simulink model "Malha_de_Controle_Drone"  (R2016a)
settings: Solver=VariableStepAuto  SolverMode=SingleTasking  StartTime=0.0  StopTime=60  RelTol=1e-3
values from neighbouring files (symbols this model uses):
  chave_circular = 0    [Controle_LQR_ARDrone.m]    (also in Controle_LQR_Robusto_Drone.m)
  chave_oito = 1    [Controle_LQR_ARDrone.m]    (also in Controle_LQR_Robusto_Drone.m)
  Cx = 0.3    [Controle_LQR_ARDrone.m]    (also in Controle_LQR_Robusto_Drone.m; TesteDeRobustez.m = 1)
  Cy = 0.1    [Controle_LQR_ARDrone.m]    (also in Controle_LQR_Robusto_Drone.m; TesteDeRobustez.m = 3)
  fimax = 0.26    [Controle_LQR_ARDrone.m]    (also in Controle_LQR_Robusto_Drone.m = 0.45)
  g = 9.8    [Controle_LQR_ARDrone.m]    (also in Controle_LQR_Robusto_Drone.m)
  K_psi = K_psi2(:,1:2)    [Controle_LQR_ARDrone.m]    (also in Controle_LQR_Robusto_Drone.m)
  K_z = K_z2(:,1:2)    [Controle_LQR_ARDrone.m]    (also in Controle_LQR_Robusto_Drone.m)
  Kfi_y = Kfi_y2(:,1:4)    [Controle_LQR_ARDrone.m]    (also in Controle_LQR_Robusto_Drone.m)
  Ki_fi_y = Kfi_y2(:,5)    [Controle_LQR_ARDrone.m]    (also in Controle_LQR_Robusto_Drone.m)
  Ki_psi = K_psi2(:,3)    [Controle_LQR_ARDrone.m]    (also in Controle_LQR_Robusto_Drone.m)
  Ki_theta_x = Ktheta_x2(:,5)    [Controle_LQR_ARDrone.m]    (also in Controle_LQR_Robusto_Drone.m)
  Ki_z = K_z2(:,3)    [Controle_LQR_ARDrone.m]    (also in Controle_LQR_Robusto_Drone.m)
  Kpsi = 1    [Controle_LQR_ARDrone.m]    (also in Controle_LQR_Robusto_Drone.m)
  Ktheta_x = Ktheta_x2(:,1:4)    [Controle_LQR_ARDrone.m]    (also in Controle_LQR_Robusto_Drone.m)
  Kz = 1.3    [Controle_LQR_ARDrone.m]    (also in Controle_LQR_Robusto_Drone.m)
  psimax = 1.74    [Controle_LQR_ARDrone.m]    (also in Controle_LQR_Robusto_Drone.m = 5.15)
  thetamax = 0.26    [Controle_LQR_ARDrone.m]    (also in Controle_LQR_Robusto_Drone.m = 0.52)
  tpsi = 0.3    [Controle_LQR_ARDrone.m]    (also in Controle_LQR_Robusto_Drone.m; TesteDeRobustez.m = 0.4)
  tz = 0.4    [Controle_LQR_ARDrone.m]    (also in Controle_LQR_Robusto_Drone.m; TesteDeRobustez.m = 0.8)
  wfi = 4.47    [Controle_LQR_ARDrone.m]    (also in Controle_LQR_Robusto_Drone.m)
  wtheta = 4.47    [Controle_LQR_ARDrone.m]    (also in Controle_LQR_Robusto_Drone.m)
  zetafi = 0.5    [Controle_LQR_ARDrone.m]    (also in Controle_LQR_Robusto_Drone.m)
  zetatheta = 0.5    [Controle_LQR_ARDrone.m]    (also in Controle_LQR_Robusto_Drone.m)
  zmax = 1.0    (= 1)    [Controle_LQR_ARDrone.m]    (also in Controle_LQR_Robusto_Drone.m = 2)
settings Model: Creator=root  LastModifiedBy=JesseAlves
settings DebuggingCC: SFUnexpectedBacktrackingDiag=error  SFNoUnconditionalDefaultTransitionDiag=error
settings SFSimCC: SimUseLocalCustomCode=on
settings RTWCC: RTWUseLocalCustomCode=on
settings GRTTargetCC: TargetLangStandard=C99 (ISO)  GeneratePreprocessorConditionals=Use local settings
settings ConfigComp: CovMetricSettings=dwe  CovHtmlReporting=off  CovSaveCumulativeToWorkspaceVar=off  CovSaveSingleToWorkspaceVar=off  CovModelRefEnable=Off  CovExternalEMLEnable=on

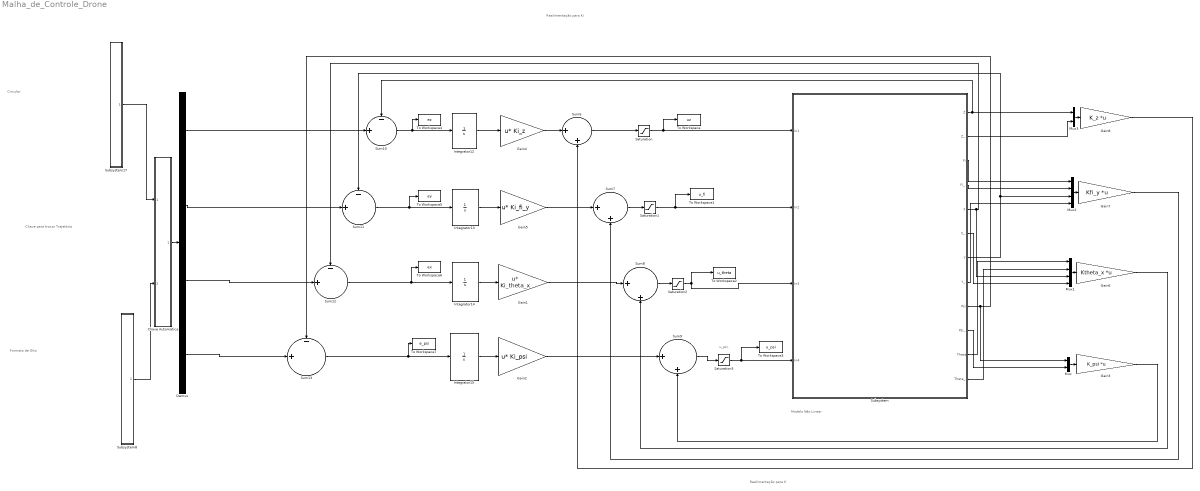
== system Malha_de_Controle_Drone ==
  note: Chave para
      | trocar Trajetória
  note: u_psi.
  note: Realimentação para Ki
  note: Modelo Não Linear
  note: Circular
  note: Formato
      | de Oito
  note: Realimentação para K
  Chave Automática : Subsystem
  Demux : Demux
  Gain1 : Gain  Gain=Ki_theta_x  Multiplication=Matrix(u*K)
  Gain2 : Gain  Gain=Ki_psi  Multiplication=Matrix(u*K)
  Gain3 : Gain  Gain=K_psi  Multiplication=Matrix(K*u)
  Gain4 : Gain  Gain=Ki_z  Multiplication=Matrix(u*K)
  Gain5 : Gain  Gain=Ki_fi_y  Multiplication=Matrix(u*K)
  Gain6 : Gain  Gain=Ktheta_x  Multiplication=Matrix(K*u)
  Gain7 : Gain  Gain=Kfi_y  Multiplication=Matrix(K*u)
  Gain8 : Gain  Gain=K_z  Multiplication=Matrix(K*u)
  Integrator{12..15} (4 alike) : Integrator
  Mux : Mux  Inputs=2
  Mux1 : Mux
  Mux2 : Mux
  Mux3 : Mux  Inputs=2
  Saturation{,1..3} (4 alike) : Saturate  UpperLimit=1  LowerLimit=-1
  Subsystem : Subsystem
  Subsystem17 : Subsystem
  Subsystem8 : Subsystem
  Sum{10..13} (4 alike) : Sum  Inputs=-+|
  Sum{6..9} (4 alike) : Sum  Inputs=|++
  To Workspace : ToWorkspace  VariableName=uz  SampleTime=-1
  To Workspace1 : ToWorkspace  VariableName=u_fi  SampleTime=-1
  To Workspace2 : ToWorkspace  VariableName=u_theta  SampleTime=-1
  To Workspace3 : ToWorkspace  VariableName=u_psi  SampleTime=-1
  To Workspace4 : ToWorkspace  VariableName=ez  SampleTime=-1
  To Workspace5 : ToWorkspace  VariableName=ey  SampleTime=-1
  To Workspace6 : ToWorkspace  VariableName=ex  SampleTime=-1
  To Workspace7 : ToWorkspace  VariableName=e_psi  SampleTime=-1
  wires:
  Sum6/1 -> Saturation/1
  Sum7/1 -> Saturation1/1
  Sum8/1 -> Saturation2/1
  Sum9/1 -> Saturation3/1
  Saturation/1 -> To Workspace/1, Subsystem/1(In1)
  Saturation1/1 -> To Workspace1/1, Subsystem/2(In2)
  Saturation2/1 -> To Workspace2/1, Subsystem/3(In3)
  Saturation3/1 -> To Workspace3/1, Subsystem/4(In4)
  Demux/1 -> Sum10/2
  Demux/2 -> Sum11/2
  Demux/3 -> Sum12/2
  Demux/4 -> Sum13/2
  Sum10/1 -> To Workspace4/1, Integrator12/1
  Integrator12/1 -> Gain4/1
  Sum11/1 -> To Workspace5/1, Integrator13/1
  Integrator13/1 -> Gain5/1
  Sum12/1 -> To Workspace6/1, Integrator14/1
  Integrator14/1 -> Gain1/1
  Integrator15/1 -> Gain2/1
  Sum13/1 -> To Workspace7/1, Integrator15/1
  Gain4/1 -> Sum6/1
  Gain5/1 -> Sum7/1
  Gain1/1 -> Sum8/1
  Gain2/1 -> Sum9/1
  Subsystem17/1(Out1) -> Chave Automática/1(In1)
  Subsystem8/1(Out1) -> Chave Automática/2(In2)
  Chave Automática/1(Out1) -> Demux/1
  Subsystem/9(Psi) -> Mux/1, Sum13/1
  Mux/1 -> Gain3/1
  Subsystem/10(Psi_.) -> Mux/2
  Gain3/1 -> Sum9/2
  Mux1/1 -> Gain6/1
  Subsystem/11(Theta) -> Mux1/1
  Subsystem/12(Theta_.) -> Mux1/2
  Subsystem/5(X) -> Sum12/1, Mux1/3
  Subsystem/6(X_.) -> Mux1/4
  Gain6/1 -> Sum8/2
  Subsystem/3(Fi) -> Mux2/1
  Subsystem/4(Fi_.) -> Mux2/2
  Subsystem/7("Y ") -> Mux2/3, Sum11/1
  Subsystem/8(Y_.) -> Mux2/4
  Mux2/1 -> Gain7/1
  Gain7/1 -> Sum7/2
  Subsystem/1(Z) -> Sum10/1, Mux3/1
  Subsystem/2("Z_. ") -> Mux3/2
  Mux3/1 -> Gain8/1
  Gain8/1 -> Sum6/2

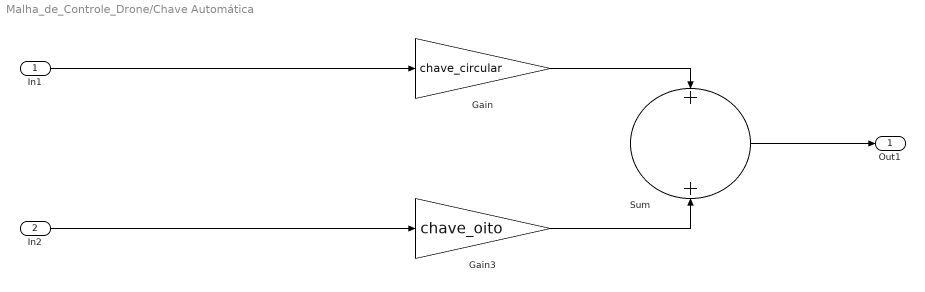
== system Malha_de_Controle_Drone/Chave Automática ==
  In1 : Inport
  In2 : Inport  Port=2
  Gain : Gain  Gain=chave_circular
  Gain3 : Gain  Gain=chave_oito
  Sum : Sum  Inputs=+|+
  Out1 : Outport
  wires:
  Sum/1 -> Out1/1
  In1/1 -> Gain/1
  In2/1 -> Gain3/1
  Gain3/1 -> Sum/2
  Gain/1 -> Sum/1

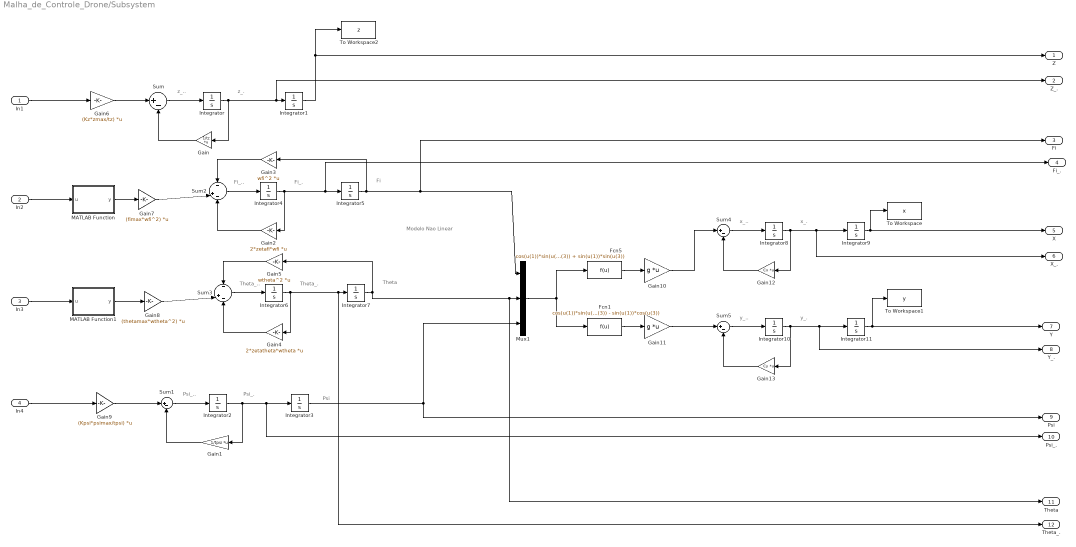
== system Malha_de_Controle_Drone/Subsystem ==
  note: Modelo Nao Linear
  note: z_..
  note: z_.
  note: Psi
  note: Psi_.
  note: Psi_..
  note: Fi
  note: Fi_.
  note: Fi_..
  note: Theta_..
  note: Theta_.
  note: Theta
  note: x_.
  note: x_..
  note: y_.
  note: y_..
  In1 : Inport
  In2 : Inport  Port=2
  In3 : Inport  Port=3
  In4 : Inport  Port=4
  Fcn1 : Fcn  Expr=cos(u(1))*sin(u(2))*sin(u(3)) - sin(u(1))*cos(u(3))
  Fcn5 : Fcn  Expr=cos(u(1))*sin(u(2))*cos(u(3)) + sin(u(1))*sin(u(3))
  Gain : Gain  Gain=1/tz  Multiplication=Matrix(K*u)
  Gain1 : Gain  Gain=1/tpsi  Multiplication=Matrix(K*u)
  Gain10 : Gain  Gain=g  Multiplication=Matrix(K*u)
  Gain11 : Gain  Gain=g  Multiplication=Matrix(K*u)
  Gain12 : Gain  Gain=Cx  Multiplication=Matrix(K*u)
  Gain13 : Gain  Gain=Cy  Multiplication=Matrix(K*u)
  Gain2 : Gain  Gain=2*zetafi*wfi  Multiplication=Matrix(K*u)
  Gain3 : Gain  Gain=wfi^2  Multiplication=Matrix(K*u)
  Gain4 : Gain  Gain=2*zetatheta*wtheta  Multiplication=Matrix(K*u)
  Gain5 : Gain  Gain=wtheta^2  Multiplication=Matrix(K*u)
  Gain6 : Gain  Gain=(Kz*zmax/tz)  Multiplication=Matrix(K*u)
  Gain7 : Gain  Gain=(fimax*wfi^2)  Multiplication=Matrix(K*u)
  Gain8 : Gain  Gain=(thetamax*wtheta^2)  Multiplication=Matrix(K*u)
  Gain9 : Gain  Gain=(Kpsi*psimax/tpsi)  Multiplication=Matrix(K*u)
  Integrator{,1..11} (12 alike) : Integrator
  MATLAB Function : MATLAB Function  TreatAsAtomicUnit=on
  MATLAB Function1 : MATLAB Function  TreatAsAtomicUnit=on
  Mux1 : Mux  Inputs=3
  Sum{,1,4..5} (4 alike) : Sum  Inputs=|+-
  Sum2 : Sum  Inputs=-|+-
  Sum3 : Sum  Inputs=-|+-
  To Workspace : ToWorkspace  VariableName=x  SampleTime=-1
  To Workspace1 : ToWorkspace  VariableName=y  SampleTime=-1
  To Workspace2 : ToWorkspace  VariableName=z  SampleTime=-1
  Z : Outport
  "Z_. " : Outport  Port=2
  Fi : Outport  Port=3
  Fi_. : Outport  Port=4
  X : Outport  Port=5
  X_. : Outport  Port=6
  "Y " : Outport  Port=7
  Y_. : Outport  Port=8
  Psi : Outport  Port=9
  Psi_. : Outport  Port=10
  Theta : Outport  Port=11
  Theta_. : Outport  Port=12
  wires:
  Integrator11/1 -> To Workspace1/1, "Y "/1
  Gain11/1 -> Sum5/1
  Gain8/1 -> Sum3/2
  Gain4/1 -> Sum3/3
  Sum5/1 -> Integrator10/1
  Sum2/1 -> Integrator4/1
  MATLAB Function1/1(y) -> Gain8/1
  Sum3/1 -> Integrator6/1
  Gain/1 -> Sum/2
  Gain7/1 -> Sum2/2
  Gain6/1 -> Sum/1
  Sum4/1 -> Integrator8/1
  Integrator1/1 -> To Workspace2/1, Z/1
  Fcn5/1 -> Gain10/1
  Integrator3/1 -> Psi/1, Mux1/3
  Integrator5/1 -> Fi/1, Mux1/1, Gain3/1
  Fcn1/1 -> Gain11/1
  Integrator4/1 -> Fi_./1, Integrator5/1, Gain2/1
  Gain5/1 -> Sum3/1
  Integrator2/1 -> Psi_./1, Integrator3/1, Gain1/1
  Integrator/1 -> "Z_. "/1, Integrator1/1, Gain/1
  Gain1/1 -> Sum1/2
  Integrator6/1 -> Theta_./1, Integrator7/1, Gain4/1
  Gain2/1 -> Sum2/3
  Gain3/1 -> Sum2/1
  Integrator9/1 -> To Workspace/1, X/1
  Gain10/1 -> Sum4/1
  Integrator10/1 -> Y_./1, Integrator11/1, Gain13/1
  Integrator7/1 -> Theta/1, Mux1/2, Gain5/1
  Gain13/1 -> Sum5/2
  Mux1/1 -> Fcn1/1, Fcn5/1
  Gain12/1 -> Sum4/2
  Sum1/1 -> Integrator2/1
  Gain9/1 -> Sum1/1
  Sum/1 -> Integrator/1
  MATLAB Function/1(y) -> Gain7/1
  Integrator8/1 -> X_./1, Integrator9/1, Gain12/1
  In1/1 -> Gain6/1
  In2/1 -> MATLAB Function/1(u)
  In3/1 -> MATLAB Function1/1(u)
  In4/1 -> Gain9/1

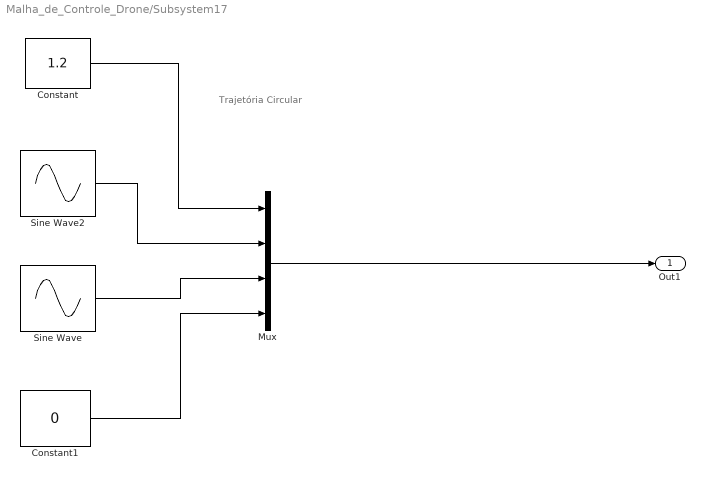
== system Malha_de_Controle_Drone/Subsystem17 ==
  note: Trajetória Circular
  Constant : Constant  Value=1.2
  Constant1 : Constant  Value=0
  Mux : Mux
  Sine Wave : Sin  Frequency=0.8  SampleTime=0
  Sine Wave2 : Sin  Frequency=0.8  Phase=pi/2  SampleTime=0
  Out1 : Outport
  wires:
  Mux/1 -> Out1/1
  Constant/1 -> Mux/1
  Sine Wave2/1 -> Mux/2
  Sine Wave/1 -> Mux/3
  Constant1/1 -> Mux/4

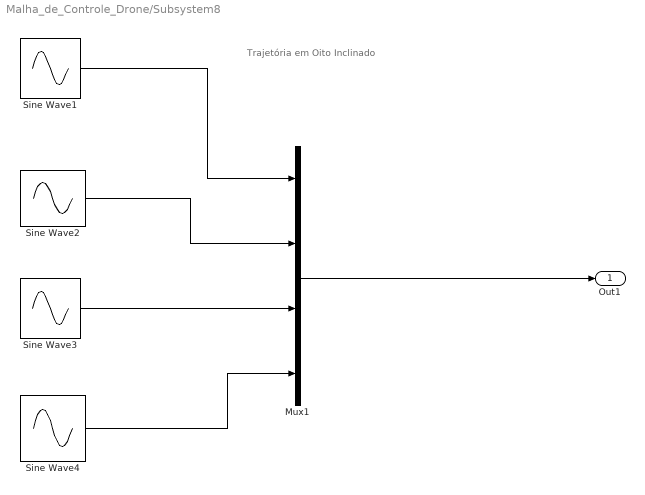
== system Malha_de_Controle_Drone/Subsystem8 ==
  note: Trajetória em Oito Inclinado
  Mux1 : Mux
  Sine Wave1 : Sin  Amplitude=0.5  Bias=1.2  Frequency=0.4  SampleTime=0
  Sine Wave2 : Sin  Frequency=0.4  SampleTime=0
  Sine Wave3 : Sin  Amplitude=0.5  Frequency=0.8  SampleTime=0
  Sine Wave4 : Sin  Amplitude=-pi/6  Frequency=0.4  SampleTime=0
  Out1 : Outport
  wires:
  Mux1/1 -> Out1/1
  Sine Wave1/1 -> Mux1/1
  Sine Wave2/1 -> Mux1/2
  Sine Wave3/1 -> Mux1/3
  Sine Wave4/1 -> Mux1/4

== matlab function Malha_de_Controle_Drone/Subsystem/MATLAB Function1 ==
  data: u input; y output
% ==> Funcao para calcular valor de K_fi
function y = k_theta(u)
    k_theta_min = 1;
    k_theta_max = 2;
    
    if abs(u) > 0.5
        u = k_theta_min*u;
    else       
        u = k_theta_max*u;
    end
y = u;

== matlab function Malha_de_Controle_Drone/Subsystem/MATLAB Function ==
  data: u input; y output
% ==> Funcao para calcular valor de K_fi
function y = k_fi(u)
    k_fi_min = 1;
    k_fi_max = 2;
    
    if abs(u) > 0.5
        u = k_fi_min*u;
    else       
        u = k_fi_max*u;
    end
y = u;
